simulink model "MCP_phase3_compensator_reduced"  (R2020a)
settings: Solver=VariableStepAuto  StartTime=0.0  StopTime=600  RelTol=1e-3
values from neighbouring files (symbols this model uses):
  h1_eq = 11.4    [Four_Tank.m]    (also in Four_Tank_phase3_LQR.m; Four_Tank_phase3_nonlinear.m; MCP_phase3_observers.m)
  h2_eq = 11.6    [Four_Tank.m]    (also in Four_Tank_phase3_LQR.m; Four_Tank_phase3_nonlinear.m; MCP_phase3_observers.m)
  h3_eq = 5.3    [Four_Tank.m]    (also in Four_Tank_phase3_LQR.m; Four_Tank_phase3_nonlinear.m = real(double(answer.h3)); MCP_phase3_observers.m)
  h4_eq = 4    [Four_Tank.m]    (also in Four_Tank_phase3_LQR.m; Four_Tank_phase3_nonlinear.m = real(double(answer.h4)); MCP_phase3_observers.m)
  v1_eq = 0.5    [Four_Tank.m]    (also in Four_Tank_phase3_LQR.m; Four_Tank_phase3_nonlinear.m = real(double(answer.v1)); MCP_phase3_observers.m)
  v2_eq = 0.5    [Four_Tank.m]    (also in Four_Tank_phase3_LQR.m; Four_Tank_phase3_nonlinear.m = real(double(answer.v2)); MCP_phase3_observers.m)
settings Model: Creator=rafiee  LastModifiedBy=Lenovo
settings DataIOCC: ReturnWorkspaceOutputs=off
settings DebuggingCC: ArithmeticOperatorsInVariantConditions=warning
settings SFSimCC: SimUseLocalCustomCode=off  CustomCodeUndefinedFunction=UseInterfaceOnly
settings RTWCC: RTWUseLocalCustomCode=off
settings CodeAppCC: StateflowObjectComments=on

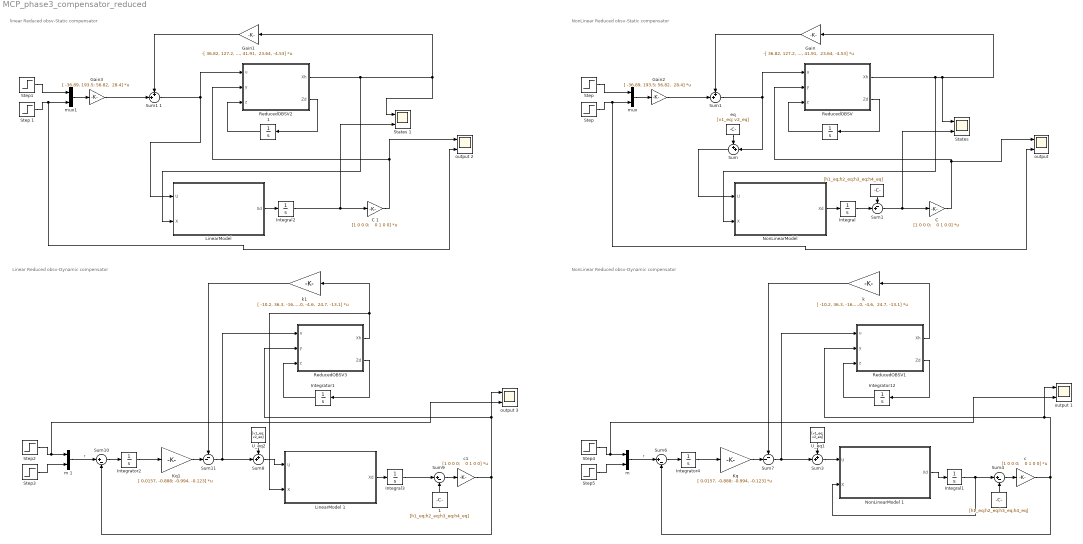
== system MCP_phase3_compensator_reduced ==
  note: NonLinear Reduced obsv-Static compensator
  note: NonLinear Reduced obsv-Dynamic compensator
  note: linear Reduced obsv-Static compensator
  note: Linear Reduced obsv-Dynamic compensator
  " " : Constant  Value=[h1_eq;h2_eq;h3_eq;h4_eq]
  "  " : Integrator  InitialCondition=[0;0]
  "     " : Constant  Value=[h1_eq;h2_eq;h3_eq;h4_eq]
  "     1" : Constant  Value=[h1_eq;h2_eq;h3_eq;h4_eq]
  "  1" : Integrator  InitialCondition=[1;1]
  " States " : Scope  NumInputPorts=2
  " States 1" : Scope  NumInputPorts=2
  "C " : Gain  Gain=|  Multiplication=Matrix(K*u)
      | [1 0 0 0;
      |    0 1 0 0]
  C 1 : Gain  Gain=|  Multiplication=Matrix(K*u)
      | [1 0 0 0;
      |    0 1 0 0]
  Gain : Gain  Gain="-[ 36.82, 127.2, -58.99, 57.97; 31.33, 41.91,  23.64, -4.53]"  Multiplication=Matrix(K*u)
  Gain1 : Gain  Gain="-[ 36.82, 127.2, -58.99, 57.97; 31.33, 41.91,  23.64, -4.53]"  Multiplication=Matrix(K*u)
  Gain2 : Gain  Gain="[ -36.89, 193.5; 56.82,  28.4]"  Multiplication=Matrix(K*u)
  Gain3 : Gain  Gain="[ -36.89, 193.5; 56.82,  28.4]"  Multiplication=Matrix(K*u)
  Integral : Integrator  InitialCondition=[h1_eq+0.1; h2_eq+0.1; h3_eq; h4_eq]
  Integral1 : Integrator  InitialCondition=[h1_eq+0.1; h2_eq+0.1; h3_eq; h4_eq]
  Integral2 : Integrator  InitialCondition=[0.5;0.5;05;0.5]
  Integral3 : Integrator  InitialCondition=[h1_eq; h2_eq; h3_eq; h4_eq]
  Integrator1 : Integrator  InitialCondition=[0;0]
  Integrator12 : Integrator  InitialCondition=[0;0]
  Integrator2 : Integrator
  Integrator4 : Integrator
  Kq : Gain  Gain=[ 0.0157, -0.888; -0.994, -0.123]  Multiplication=Matrix(K*u)
  Kq1 : Gain  Gain=[ 0.0157, -0.888; -0.994, -0.123]  Multiplication=Matrix(K*u)
  "LinearModel " : MATLAB Function  TreatAsAtomicUnit=on
  LinearModel 1 : MATLAB Function  TreatAsAtomicUnit=on
  "NonLinearModel " : MATLAB Function  TreatAsAtomicUnit=on
  NonLinearModel 1 : MATLAB Function  TreatAsAtomicUnit=on
  ReducedOBSV : MATLAB Function  TreatAsAtomicUnit=on
  ReducedOBSV1 : MATLAB Function  TreatAsAtomicUnit=on
  ReducedOBSV2 : MATLAB Function  TreatAsAtomicUnit=on
  ReducedOBSV3 : MATLAB Function  TreatAsAtomicUnit=on
  Step{,1..5} (6 alike) : Step  SampleTime=0
  "Step " : Step  SampleTime=0
  Step 1 : Step  SampleTime=0
  Sum : Sum  Inputs=++|
  Sum1 : Sum  Inputs=-+|
  "Sum1 " : Sum  Inputs=++|
  Sum1 1 : Sum  Inputs=++|
  Sum{4,6,9..10} (4 alike) : Sum  Inputs=|+-
  Sum11 : Sum  Inputs=--|
  Sum3 : Sum  Inputs=++|
  Sum7 : Sum  Inputs=--|
  Sum8 : Sum  Inputs=++|
  U_eq1 : Constant  Value=[v1_eq; v2_eq]
  U_eq2 : Constant  Value=[v1_eq; v2_eq]
  c : Gain  Gain=|  Multiplication=Matrix(K*u)
      | [1 0 0 0;
      |    0 1 0 0]
  c1 : Gain  Gain=|  Multiplication=Matrix(K*u)
      | [1 0 0 0;
      |    0 1 0 0]
  eq : Constant  Value=[v1_eq; v2_eq]
  k : Gain  Gain="[ -10.2, 36.3, -16.5,  24.5; 41.0, -4.6,  24.7, -13.1]"  Multiplication=Matrix(K*u)
  k1 : Gain  Gain="[ -10.2, 36.3, -16.5,  24.5; 41.0, -4.6,  24.7, -13.1]"  Multiplication=Matrix(K*u)
  "m " : Concatenate
  m 1 : Concatenate
  mux : Concatenate
  mux1 : Concatenate
  output {,1..3} (4 alike) : Scope  NumInputPorts=2
  wires:
  Integral/1 -> Sum1/2
  Gain2/1 -> "Sum1 "/2
  "  "/1 -> ReducedOBSV/3(z)
  mux/1 -> Gain2/1
  " "/1 -> Sum1/1
  Sum/1 -> "NonLinearModel "/1(U)
  eq/1 -> Sum/1
  Step/1 -> mux/1
  Gain/1 -> "Sum1 "/1
  ReducedOBSV/2(Zd) -> "  "/1
  "C "/1 -> ReducedOBSV/2(y), "output "/1
  "Sum1 "/1 -> Sum/2, ReducedOBSV/1(u)
  ReducedOBSV/1(Xh) -> "NonLinearModel "/2(X), Gain/1, " States "/1
  "Step "/1 -> "output "/2, mux/2
  "NonLinearModel "/1(Xd) -> Integral/1
  Sum1/1 -> " States "/2, "C "/1
  c/1 -> output 1/1, ReducedOBSV1/2(y), Sum6/2
  Step5/1 -> "m "/2
  Sum6/1 -> Integrator4/1
  Kq/1 -> Sum7/2
  Integral1/1 -> NonLinearModel 1/2(X), Sum4/1
  "     "/1 -> Sum4/2
  ReducedOBSV1/2(Zd) -> Integrator12/1
  ReducedOBSV1/1(Xh) -> k/1
  NonLinearModel 1/1(Xd) -> Integral1/1
  U_eq1/1 -> Sum3/1
  Integrator12/1 -> ReducedOBSV1/3(z)
  Step4/1 -> output 1/2, "m "/1
  Integrator4/1 -> Kq/1
  Sum3/1 -> NonLinearModel 1/1(U)
  Sum4/1 -> c/1
  k/1 -> Sum7/1
  Sum7/1 -> ReducedOBSV1/1(u), Sum3/2
  "m "/1 -> Sum6/1  "r"
  Integral2/1 -> C 1/1, " States 1"/2
  "LinearModel "/1(Xd) -> Integral2/1
  Step 1/1 -> output 2/2, mux1/2
  ReducedOBSV2/1(Xh) -> "LinearModel "/2(X), Gain1/1, " States 1"/1
  C 1/1 -> ReducedOBSV2/2(y), output 2/1
  ReducedOBSV2/2(Zd) -> "  1"/1
  Gain1/1 -> Sum1 1/1
  Step1/1 -> mux1/1
  Sum1 1/1 -> "LinearModel "/1(U), ReducedOBSV2/1(u)
  mux1/1 -> Gain3/1
  "  1"/1 -> ReducedOBSV2/3(z)
  Gain3/1 -> Sum1 1/2
  m 1/1 -> Sum10/1  "r"
  Sum11/1 -> Sum8/2, ReducedOBSV3/1(u)
  k1/1 -> Sum11/1
  Sum9/1 -> c1/1
  Sum8/1 -> LinearModel 1/1(U)
  Integrator2/1 -> Kq1/1
  Step2/1 -> output 3/2, m 1/1
  Integrator1/1 -> ReducedOBSV3/3(z)
  U_eq2/1 -> Sum8/1
  LinearModel 1/1(Xd) -> Integral3/1
  ReducedOBSV3/2(Zd) -> Integrator1/1
  "     1"/1 -> Sum9/2
  Integral3/1 -> Sum9/1
  Kq1/1 -> Sum11/2
  Sum10/1 -> Integrator2/1
  Step3/1 -> m 1/2
  c1/1 -> Sum10/2, ReducedOBSV3/2(y), output 3/1
  ReducedOBSV3/1(Xh) -> k1/1, LinearModel 1/2(X)

== matlab function MCP_phase3_compensator_reduced/ReducedOBSV1 ==
  data: Xh output size=[4,1]; u input size=[2,1]; Zd output size=[2,1]; y input size=[2,1]; z input size=[2,1]
function [Xh, Zd]= Obsv_Reduced(u , y, z)
% System main Matrices
B = [ 0.00306,      0;
       0, 0.0035;
       0, 0.0065;
 0.00714,      0];


 C = [ 1.0,   0, 0, 0;
   0, 1.0, 0, 0];

% Observer Matrices
F = diag([-0.4,-0.45]);

T = [ 2.62,     0, -0.205,     0;
    0, -2.32,      0, 0.195];


L = [ 1.0,    0;
   0, -1.0];

Zd = F*z + T*B*u + L*y;
Xh = ([C;T]^-1)*[y;z];
end

== matlab function MCP_phase3_compensator_reduced/NonLinearModel 1 ==
  data: U input; Xd output; X input
function Xd = NonlinearModel(U, X)

A = [730 730 730 730];
a = [2.10 2.14 2.2 2.3];
g = 981;
y = [0.3 0.35];
k = [7.45 7.30];

v1 = U(1);
v2 = U(2);

h1 = X(1);
h2 = X(2);
h3 = X(3);
h4 = X(4);

h1_d = -a(1)/A(1)*sqrt(2*g*h1)+a(3)/A(1)*sqrt(2*g*h3)+y(1)*k(1)/A(1)*v1;
h2_d = -a(2)/A(2)*sqrt(2*g*h2)+a(4)/A(2)*sqrt(2*g*h4)+y(2)*k(2)/A(2)*v2;
h3_d = -a(3)/A(3)*sqrt(2*g*h3)+(1 - y(2))*k(2)/A(3)*v2;
h4_d = -a(4)/A(4)*sqrt(2*g*h4)+(1 - y(1))*k(1)/A(4)*v1;

Xd = [h1_d;h2_d;h3_d;h4_d];

== matlab function MCP_phase3_compensator_reduced/LinearModel  ==
  data: U input; Xd output; X input
function Xd = linear_system(U, X)

A = [ -0.01887,        0,  0.02848,        0;
        0, -0.01906,        0,  0.03557;
        0,        0, -0.02848,        0;
        0,        0,        0, -0.03557];
    
B = [ 0.003062,      0;
         0, 0.0035;
        0, 0.0065;
 0.007144,      0];

Xd = A * X + B * U;

== matlab function MCP_phase3_compensator_reduced/ReducedOBSV2 ==
  data: Xh output size=[4,1]; u input size=[2,1]; Zd output size=[2,1]; y input size=[2,1]; z input size=[2,1]
function [Xh, Zd]= Obsv_Reduced(u , y, z)
% System main Matrices
B = [ 0.00306,      0;
       0, 0.0035;
       0, 0.0065;
 0.00714,      0];


 C = [ 1.0,   0, 0, 0;
   0, 1.0, 0, 0];

% Observer Matrices
F = diag([-0.4,-0.45]);

T = [ 2.62,     0, -0.205,     0;
    0, -2.32,      0, 0.195];


L = [ 1.0,    0;
   0, -1.0];

Zd = F*z + T*B*u + L*y;
Xh = ([C;T]^-1)*[y;z];
end

== matlab function MCP_phase3_compensator_reduced/LinearModel 1 ==
  data: U input; Xd output; X input
function Xd = linear_system(U, X)

A = [ -0.01887,        0,  0.02848,        0;
        0, -0.01906,        0,  0.03557;
        0,        0, -0.02848,        0;
        0,        0,        0, -0.03557];
    
B = [ 0.003062,      0;
         0, 0.0035;
        0, 0.0065;
 0.007144,      0];

Xd = A * X + B * U;

== matlab function MCP_phase3_compensator_reduced/ReducedOBSV3 ==
  data: Xh output size=[4,1]; u input size=[2,1]; Zd output size=[2,1]; y input size=[2,1]; z input size=[2,1]
function [Xh, Zd]= Obsv_Reduced(u , y, z)
% System main Matrices
B = [ 0.00306,      0;
       0, 0.0035;
       0, 0.0065;
 0.00714,      0];


 C = [ 1.0,   0, 0, 0;
   0, 1.0, 0, 0];

% Observer Matrices
F = diag([-0.4,-0.45]);

T = [ 2.62,     0, -0.205,     0;
    0, -2.32,      0, 0.195];


L = [ 1.0,    0;
   0, -1.0];

Zd = F*z + T*B*u + L*y;
Xh = ([C;T]^-1)*[y;z];
end

== matlab function MCP_phase3_compensator_reduced/ReducedOBSV ==
  data: Xh output size=[4,1]; u input size=[2,1]; Zd output size=[2,1]; y input size=[2,1]; z input size=[2,1]
function [Xh, Zd]= Obsv_Reduced(u , y, z)
% System main Matrices
B = [ 0.00306,      0;
       0, 0.0035;
       0, 0.0065;
 0.00714,      0];


 C = [ 1.0,   0, 0, 0;
   0, 1.0, 0, 0];

% Observer Matrices
F = diag([-0.4,-0.45]);

T = [ 2.62,     0, -0.205,     0;
    0, -2.32,      0, 0.195];


L = [ 1.0,    0;
   0, -1.0];

Zd = F*z + T*B*u + L*y;
Xh = ([C;T]^-1)*[y;z];
end

== matlab function MCP_phase3_compensator_reduced/NonLinearModel  ==
  data: U input; Xd output; X input
function Xd = NonlinearModel(U, X)

A = [730 730 730 730];
a = [2.10 2.14 2.2 2.3];
g = 981;
y = [0.3 0.35];
k = [7.45 7.30];

v1 = U(1);
v2 = U(2);

h1 = X(1);
h2 = X(2);
h3 = X(3);
h4 = X(4);

h1_d = -a(1)/A(1)*sqrt(2*g*h1)+a(3)/A(1)*sqrt(2*g*h3)+y(1)*k(1)/A(1)*v1;
h2_d = -a(2)/A(2)*sqrt(2*g*h2)+a(4)/A(2)*sqrt(2*g*h4)+y(2)*k(2)/A(2)*v2;
h3_d = -a(3)/A(3)*sqrt(2*g*h3)+(1 - y(2))*k(2)/A(3)*v2;
h4_d = -a(4)/A(4)*sqrt(2*g*h4)+(1 - y(1))*k(1)/A(4)*v1;

Xd = [h1_d;h2_d;h3_d;h4_d];
